simulink model "large_scale_autosar_swc_expfcns"  (R2021a)
settings: Solver=FixedStepDiscrete  StartTime=0.0  StopTime=20  FixedStep=1  MaxStep=.0001  RelTol=1e-3  EnableMultiTasking=on
undefined symbols (not defined in the file): DiscIntNeverNeededParam
(part 3 of 3)

== system large_scale_autosar_swc_expfcns/Runnable98_subsystem ==
  u : Inport
  function : TriggerPort  TriggerType=function-call  VariantControl=Variant  SampleTimeType=periodic  SampleTime=-1
  gain : Gain  Gain=-1  ParamDataTypeStr=int8  OutDataTypeStr=int8
  y : Outport  InitialOutput=0  VectorParamsAs1DForOutWhenUnconnected=off
  y1 : Outport  Port=2  VectorParamsAs1DForOutWhenUnconnected=off
  wires:
  u/1 -> gain/1
  gain/1 -> y/1, y1/1

== system large_scale_autosar_swc_expfcns/Runnable99_subsystem ==
  u : Inport
  function : TriggerPort  TriggerType=function-call  VariantControl=Variant  SampleTimeType=periodic  SampleTime=-1
  gain : Gain  Gain=-1  ParamDataTypeStr=int8  OutDataTypeStr=int8
  y : Outport  InitialOutput=0  VectorParamsAs1DForOutWhenUnconnected=off
  y1 : Outport  Port=2  VectorParamsAs1DForOutWhenUnconnected=off
  wires:
  u/1 -> gain/1
  gain/1 -> y/1, y1/1

== system large_scale_autosar_swc_expfcns/Runnable9_subsystem ==
  u : Inport
  function : TriggerPort  TriggerType=function-call  VariantControl=Variant  SampleTimeType=periodic  SampleTime=-1
  gain : Gain  Gain=-1  ParamDataTypeStr=int8  OutDataTypeStr=int8
  y : Outport  InitialOutput=0  VectorParamsAs1DForOutWhenUnconnected=off
  y1 : Outport  Port=2  VectorParamsAs1DForOutWhenUnconnected=off
  wires:
  u/1 -> gain/1
  gain/1 -> y/1, y1/1

== system large_scale_autosar_swc_expfcns/Runnable1_subsystem/Subsystem ==
  In1 : Inport
  In2 : Inport  Port=2
  Enable : EnablePort
  Add : Sum
  Adder : Outport  VectorParamsAs1DForOutWhenUnconnected=off
  wires:
  In2/1 -> Add/2
  In1/1 -> Add/1
  Add/1 -> Adder/1
